simulink model "NeuroControlExamen"  (R2023b)
settings: Solver=VariableStepAuto  StartTime=0.0  StopTime=10.0  RelTol=1e-3
(part 3 of 3)

== matlab function NeuroControlExamen/MATLAB Function3 ==
  data: omega_hat_d output; q input; qd input
function omega_hat_d  = fcn(q,qd)

alpha = diag([5 5 5]);
Gamma = diag([1 1 1 1 1 1 1 1 1 1 1 1 1 1 1])*50;

q_deseada = [0.3;0.4;0.5];
qd_deseada = [0;0;0];
difq = q-q_deseada;
difqd = qd-qd_deseada;

S = difqd+alpha*difq;

phi = [difq; difqd; q_deseada; qd_deseada; S];

omega_hat_d = -Gamma*phi*S.';
